simulink model "current_mode_model"  (R2024b)
settings: Solver=VariableStepAuto  StartTime=0.0  StopTime=0.8  FixedStep=1e-6  RelTol=1e-3
InitFcn:
  | tao = 0.516;
  | J = 4.943e-4;
  | b = J/tao;
  | Kt = 0.164;
  | R = 0.106/2;
  | L = (0.428e-3)/2;
  | pn = 2;
  | 
  | TL = 0.3;
  | wL = 800/(30/pi);
  | wH = 1300/(30/pi);
  | IH = (J/tao*wH+TL)/Kt;
  | IL = (J/tao*wL+TL)/Kt;
undefined symbols (not defined in the file or in its folder): DiscIntNeverNeededParam
libraries: spsPermanentMagnetSynchronousMachineLib x1, spsDCVoltageSourceLib x1, spsGroundLib x1, spsUniversalBridgeLib x1, sps_lib x1

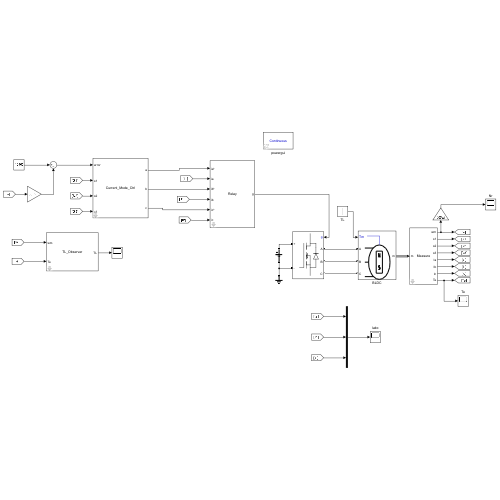
[thumbnail: Simulink's stored preview of the top-level diagram]
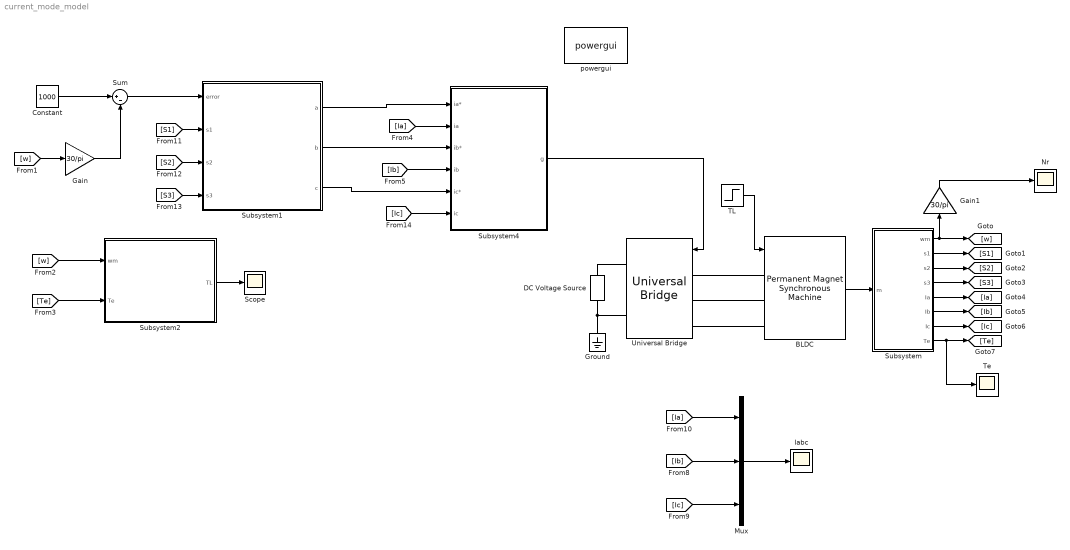
== system current_mode_model ==
  BLDC : spsPermanentMagnetSynchronousMachineLib/Permanent Magnet Synchronous Machine  NbPhases=3  FluxDistribution=Trapezoidal  RotorType=Round  MechanicalLoad=Torque Tm  PresetModel=No  ShowDetailedParameters=on  MeasurementBus=off  Resistance=R  Inductance=L  dqInductances=[8.5e-3,8.5e-3]  La=0.000395  MachineConstant=Torque Constant (N.m / A_peak)  Flux=0.041  VoltageCst=17.174  TorqueCst=Kt  Flat=120  Mechanical=[J b pn 0]  PolePairs=4  InitialConditions=[0,0, 0,0]  InitialConditions5ph=[0 0 0 0 0 0]  RefAngle=Aligned with phase A axis (original Park)  IterativeDiscreteModel=Trapezoidal non iterative  TsBlock=-1  TsPowergui=0
  Constant : Constant  Value=1000
  DC Voltage Source : spsDCVoltageSourceLib/DC Voltage Source  Amplitude=50  Measurements=None
  Gain : Gain  Gain=30/pi
  Gain1 : Gain  Gain=30/pi
  Ground : spsGroundLib/Ground  LConnTagsString=a
  Iabc : Scope
  Mux : Mux  Inputs=3
  Nr : Scope
  Scope : Scope
  Subsystem : Subsystem
  Subsystem1 : Subsystem  mask{Ts=1/(800), IH=2.72, IL=2.31}
      mask prompts: Ts "Ts : sample period"; IH "IH : high current"; IL "IL : low current"
  Subsystem2 : Subsystem  mask{Ts=1/(1e3), IH=2.72, IL=2.31}
      mask prompts: Ts "Ts : sample period"; IH "IH : high current"; IL "IL : low current"
  Subsystem4 : Subsystem  mask{band=0.15}
      mask prompts: band "band : bandwidth"
  Sum : Sum  Inputs=|+-
  TL : Step  Time=0.1  Before=0.1  After=TL  SampleTime=0
  Te : Scope
  Universal Bridge : spsUniversalBridgeLib/Universal Bridge  Arms=3  SnubberResistance=1e5  SnubberCapacitance=inf  Device=MOSFET / Diodes  Ron=1e-3  Lon=0  ForwardVoltages="[  0  0  ]"  ForwardVoltage=0  GTOparameters=[ 10e-6 , 20e-6 ]  IGBTparameters=[ 1e-6 , 2e-6 ]  Measurements=None  Measurements_2=None  converterType=Rectifier
  powergui : sps_lib/powergui  Priority=1  SimulationMode=Continuous  SampleTime=1e-6  frequency=60  Iterations=50  frequencyindice=0  Pbase=100e6  ErrMax=1e-4  UnitsV=kV  UnitsW=MW  buscounter=0  FunctionMessages=off  echomessages=off  EnableUseOfTLC=off  CurrentSourceSwitches=off  DisableSnubberDevices=off  DisableRonSwitches=off  DisableVfSwitches=off  DisplayEquations=off  AutomaticDiscreteSolvers=off  SolverType=Tustin/Backward Euler (TBE)  Interpol=off  ExternalGateDelay=off  methode=off  Ts=100  x0status=blocks  SPID=on  SwTol=0  HookPort=off  NonlinearTolerance=1e-4  nMaxIteration=100  ContinueOnMaxIteration=off  RestoreLinks=warning  ResistiveCurrentMeasurement=off  Frange=[0:2:500]  Ylog=off  Xlog=on  ShowGrid=off  save=off  variable=ZData  structure=0  ZoomFFT=off  StartTime=0.0  cycles=1  DisplayStyle=1  fundamental=60  FreqAxis=off  MaxFrequency=1000  frequencyindicesteady=1  RmsSteady=1  display=off
  wires:
  Mux/1 -> Iabc/1
  [Ic] -> Mux/3
  [Ia] -> Mux/1
  [Ib] -> Mux/2
  TL/1 -> BLDC/1
  BLDC/1 -> Subsystem/1(m)
  Subsystem/6(Ib) -> [Ib]
  Subsystem/2(s1) -> [S1]
  Subsystem/5(Ia) -> [Ia]
  Subsystem/7(Ic) -> [Ic]
  Subsystem/8(Te) -> Te/1, [Te]
  Subsystem/1(wm) -> Gain1/1, [w]
  Subsystem/3(s2) -> [S2]
  Gain1/1 -> Nr/1
  Subsystem/4(s3) -> [S3]
  Subsystem4/1(g) -> Universal Bridge/1
  [S3] -> Subsystem1/4(s3)
  Subsystem1/1(a) -> Subsystem4/1(ia*)
  [S2] -> Subsystem1/3(s2)
  [S1] -> Subsystem1/2(s1)
  [Ia] -> Subsystem4/2(ia)
  [Ib] -> Subsystem4/4(ib)
  Subsystem1/2(b) -> Subsystem4/3(ib*)
  Subsystem1/3(c) -> Subsystem4/5(ic*)
  [Ic] -> Subsystem4/6(ic)
  Constant/1 -> Sum/1
  [w] -> Gain/1
  Gain/1 -> Sum/2
  Sum/1 -> Subsystem1/1(error)
  [w] -> Subsystem2/1(wm)
  [Te] -> Subsystem2/2(Te)
  Subsystem2/1(TL) -> Scope/1
  connections:
  Universal Bridge/LConn3 -- BLDC/LConn3
  Universal Bridge/LConn2 -- BLDC/LConn2
  Universal Bridge/LConn1 -- BLDC/LConn1
  DC Voltage Source/RConn1 -- Universal Bridge/RConn1
  DC Voltage Source/LConn1 -- Ground/LConn1 -- Universal Bridge/RConn2

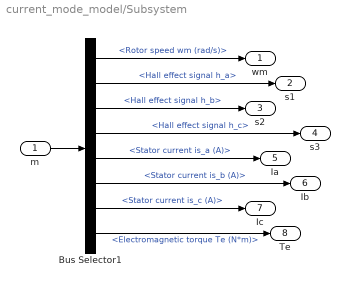
== system current_mode_model/Subsystem ==
  m : Inport
  Bus Selector1 : BusSelector  OutputSignals=Rotor speed wm (rad/s),Hall effect signal h_a,Hall effect signal h_b,Hall effect signal h_c,Stator current is_a (A),Stator current is_b (A),Stator current is_c (A),Electromagnetic torque Te (N*m)
  wm : Outport
  s1 : Outport  Port=2
  s2 : Outport  Port=3
  s3 : Outport  Port=4
  Ia : Outport  Port=5
  Ib : Outport  Port=6
  Ic : Outport  Port=7
  Te : Outport  Port=8
  wires:
  m/1 -> Bus Selector1/1
  Bus Selector1/5 -> Ia/1  "<Stator current is_a (A)>"
  Bus Selector1/8 -> Te/1  "<Electromagnetic torque Te (N*m)>"
  Bus Selector1/6 -> Ib/1  "<Stator current is_b (A)>"
  Bus Selector1/7 -> Ic/1  "<Stator current is_c (A)>"
  Bus Selector1/1 -> wm/1  "<Rotor speed wm (rad/s)>"
  Bus Selector1/2 -> s1/1  "<Hall effect signal h_a>"
  Bus Selector1/3 -> s2/1  "<Hall effect signal h_b>"
  Bus Selector1/4 -> s3/1  "<Hall effect signal h_c>"

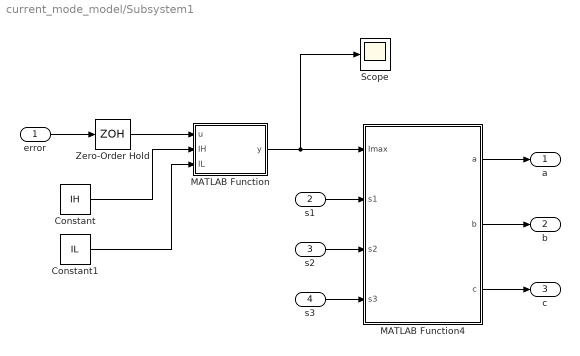
== system current_mode_model/Subsystem1 ==
  error : Inport
  s1 : Inport  Port=2
  s2 : Inport  Port=3
  s3 : Inport  Port=4
  Constant : Constant  Value=IH
  Constant1 : Constant  Value=IL
  MATLAB Function : MATLAB Function  TreatAsAtomicUnit=on
  MATLAB Function4 : MATLAB Function  TreatAsAtomicUnit=on
  Scope : Scope
  Zero-Order Hold : ZeroOrderHold  SampleTime=Ts
  a : Outport
  b : Outport  Port=2
  c : Outport  Port=3
  wires:
  error/1 -> Zero-Order Hold/1
  MATLAB Function/1(y) -> Scope/1, MATLAB Function4/1(Imax)
  Zero-Order Hold/1 -> MATLAB Function/1(u)
  Constant/1 -> MATLAB Function/2(IH)
  Constant1/1 -> MATLAB Function/3(IL)
  s1/1 -> MATLAB Function4/2(s1)
  s2/1 -> MATLAB Function4/3(s2)
  s3/1 -> MATLAB Function4/4(s3)
  MATLAB Function4/1(a) -> a/1
  MATLAB Function4/2(b) -> b/1
  MATLAB Function4/3(c) -> c/1

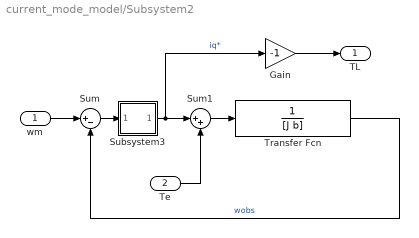
== system current_mode_model/Subsystem2 ==
  wm : Inport
  Te : Inport  Port=2
  Gain : Gain  Gain=-1
  Subsystem3 : Subsystem  mask{Ki=5000*J, Kp=5000*b, int_limit=[-30,30], out_limit=[-30,30], Ts=1/(10e3)}
      mask prompts: Ki "Ki : Integral"; Kp "Kp : Propotional"; int_limit "integral limit : [min, max]"; out_limit "output limit : [min, max]"; Ts "Ts : sample time"
  Sum : Sum  Inputs=|+-
  Sum1 : Sum  Inputs=|++
  Transfer Fcn : TransferFcn  Denominator=[J b]
  TL : Outport
  wires:
  wm/1 -> Sum/1
  Sum/1 -> Subsystem3/1(Input)
  Subsystem3/1(output) -> Gain/1, Sum1/1  "iq*"
  Sum1/1 -> Transfer Fcn/1
  Te/1 -> Sum1/2
  Transfer Fcn/1 -> Sum/2  "wobs"
  Gain/1 -> TL/1

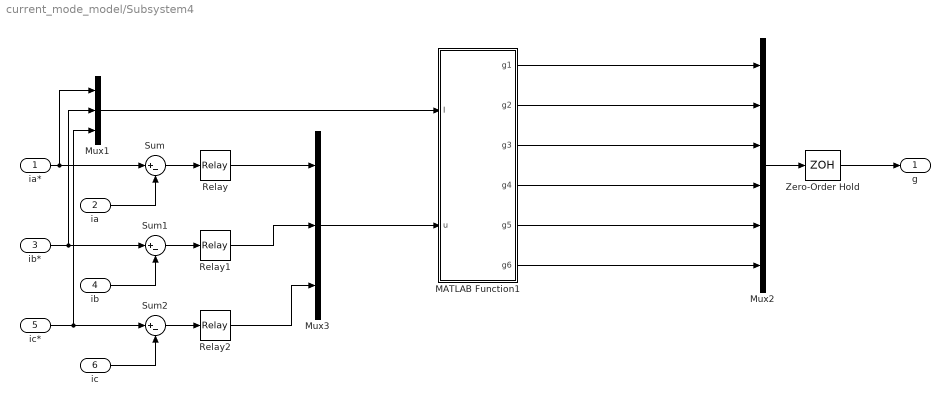
== system current_mode_model/Subsystem4 ==
  ia* : Inport
  ia : Inport  Port=2
  ib* : Inport  Port=3
  ib : Inport  Port=4
  ic* : Inport  Port=5
  ic : Inport  Port=6
  MATLAB Function1 : MATLAB Function  TreatAsAtomicUnit=on
  Mux1 : Mux  Inputs=3
  Mux2 : Mux  Inputs=6
  Mux3 : Mux  Inputs=3
  Relay : Relay  OnSwitchValue=band/2  OffSwitchValue=-band/2
  Relay1 : Relay  OnSwitchValue=band/2  OffSwitchValue=-band/2
  Relay2 : Relay  OnSwitchValue=band/2  OffSwitchValue=-band/2
  Sum : Sum  Inputs=|+-
  Sum1 : Sum  Inputs=|+-
  Sum2 : Sum  Inputs=|+-
  Zero-Order Hold : ZeroOrderHold  SampleTime=1/(500e3)
  g : Outport
  wires:
  ia*/1 -> Mux1/1, Sum/1
  ia/1 -> Sum/2
  Sum/1 -> Relay/1
  Relay/1 -> Mux3/1
  Sum1/1 -> Relay1/1
  Relay1/1 -> Mux3/2
  ib*/1 -> Mux1/2, Sum1/1
  ib/1 -> Sum1/2
  Sum2/1 -> Relay2/1
  Relay2/1 -> Mux3/3
  ic*/1 -> Sum2/1, Mux1/3
  ic/1 -> Sum2/2
  Mux1/1 -> MATLAB Function1/1(I)
  MATLAB Function1/1(g1) -> Mux2/1
  MATLAB Function1/2(g2) -> Mux2/2
  MATLAB Function1/3(g3) -> Mux2/3
  MATLAB Function1/4(g4) -> Mux2/4
  MATLAB Function1/5(g5) -> Mux2/5
  MATLAB Function1/6(g6) -> Mux2/6
  Mux3/1 -> MATLAB Function1/2(u)
  Mux2/1 -> Zero-Order Hold/1
  Zero-Order Hold/1 -> g/1

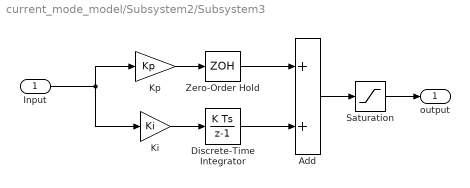
== system current_mode_model/Subsystem2/Subsystem3 ==
  Input : Inport
  Add : Sum
  Discrete-Time Integrator : DiscreteIntegrator  SampleTime=Ts  LimitOutput=on  UpperSaturationLimit=int_limit(2)  LowerSaturationLimit=int_limit(1)  ICPrevOutput=DiscIntNeverNeededParam  ICPrevScaledInput=DiscIntNeverNeededParam
  Ki : Gain  Gain=Ki
  Kp : Gain  Gain=Kp
  Saturation : Saturate  UpperLimit=out_limit(2)  LowerLimit=out_limit(1)
  Zero-Order Hold : ZeroOrderHold  SampleTime=Ts
  output : Outport
  wires:
  Input/1 -> Ki/1, Kp/1
  Ki/1 -> Discrete-Time Integrator/1
  Discrete-Time Integrator/1 -> Add/2
  Add/1 -> Saturation/1
  Saturation/1 -> output/1
  Kp/1 -> Zero-Order Hold/1
  Zero-Order Hold/1 -> Add/1

== matlab function current_mode_model/Subsystem1/MATLAB Function4 ==
function [a,b,c] = Current_Cmd(Imax,s1,s2,s3)
    states = s1*4 + s2*2 + s3*1;
    a = 0;
    b = 0;
    c = 0;
    if states == 0 || states == 7
    % error Hall signals, stop motor
        return;
    end

    %map table
    map_tab = [6, 4, 5, 2, 1, 3];
    six_commut_tab = [1,-1,0; 1,0,-1;0,1,-1;-1,1,0;-1,0,1;0,-1,1];
    if Imax > 0 %CCW, forward rotation
        index = map_tab(states);
    else %CW, reversal rotation
        index = mod(map_tab(states) - 1 + 3,6) + 1;
    end
    A = six_commut_tab(index,1);
    B = six_commut_tab(index,2);
    C = six_commut_tab(index,3);
    %produce current command
    
    if A == 0
        if B > 0
            b = Imax;
            c = -Imax;
        else
            b = -Imax;
            c = Imax;
        end
    elseif B == 0
        if A > 0
            a = Imax;
            c = -Imax;
        else
            a = -Imax;
            c = Imax;
        end
    elseif C == 0
        if A > 0
            a = Imax;
            b = -Imax;
        else
            a = -Imax;
            b = Imax;
        end
    end
end

== matlab function current_mode_model/Subsystem1/MATLAB Function ==
function y = fcn(u,IH,IL)
    if u <= 0
        y = IL;
    else
        y = IH;
    end

== matlab function current_mode_model/Subsystem4/MATLAB Function1 ==
function [g1, g2, g3, g4, g5, g6] = fcn(I, u)
if I(1) == 0 && I(2) == 0 && I(3) == 0
    u = [0,0,0,0,0,0];
elseif I(1) == 0
    if u(2) > 0
            u = [0,0,1,0,0,1];%normal operate
    else
            u = [0,0,0,1,1,0];%change sector
    end
elseif I(2) == 0
     if u(1) > 0
            u = [1,0,0,0,0,1];
     else
            u = [0,1,0,0,1,0];
     end
else
    % sector 1
     if u(1) > 0
            u = [1,0,0,1,0,0];%normal operate
     else
            u = [0,1,1,0,0,0];%normal operate
     end
end
%
g1 = u(1);
g2 = u(2);
g3 = u(3);
g4 = u(4);
g5 = u(5);
g6 = u(6);
